simulink model "AnaModelFault000"  (R2018b)
settings: Solver=VariableStepAuto  StartTime=0.0  StopTime=2  MaxStep=1e-4  RelTol=1e-3
values from neighbouring files (symbols this model uses):
  J = 0.275e-3    (= 0.000275)    [StateSpace.m]    (also in init_AnaModel003.m)
  Ki = 1    [init_AnaModel003.m]
  Kp = 0.05    [init_AnaModel003.m]
  L0 = Ll + 1.5*Lms    (= 0.00130602)    [StateSpace.m]    (also in init_AnaModel003.m)
  L1 = Ll + 1.5*Lms    [AnaModel.m]    (also in StateSpace.m = (sqrt(3)* Llm + 1.5 *Lms); init_AnaModel003.m = (sqrt(3)* Llm + 1.5 *Lms))
  L2 = (sqrt(3)/2)*Lms + Llm    [AnaModel.m]    (also in StateSpace.m = 0.0010375; init_AnaModel003.m = 0.0010375)
  P = 6    [StateSpace.m]    (also in init_AnaModel003.m)
  Phi_f = 0.03    [StateSpace.m]    (also in init_AnaModel003.m)
  rs = 1.98    [StateSpace.m]    (also in init_AnaModel003.m)
  Tm = 1    [StateSpace.m]    (also in init_AnaModel003.m)
libraries: powerlib x46, powerlib_meascontrol x9, simulink x7
(part 1 of 2)
settings Model: Creator=admin  LastModifiedBy=aeish
settings SolverCC: ZeroCrossAlgorithm=Adaptive
settings DebuggingCC: MaxConsecutiveZCsMsg=none  LibraryContextMissingDiagnostic=none
settings SFSimCC: SimUseLocalCustomCode=off
settings RTWCC: RTWUseLocalCustomCode=off

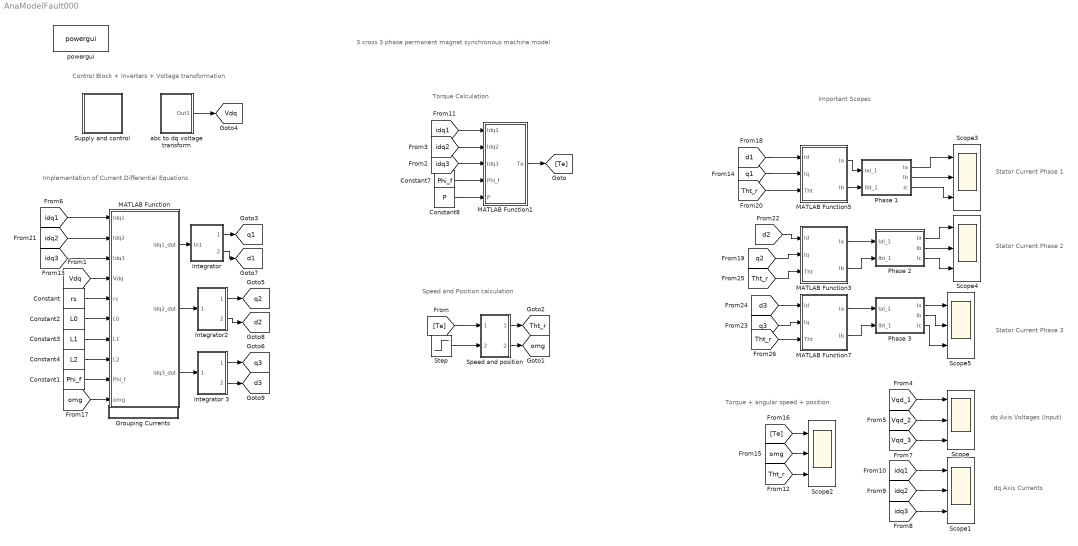
== system AnaModelFault000 ==
  note: 3 cross 3 phase permanent magnet synchronous machine model
  note: Torque + angular speed + position
  note: dq Axis Voltages (Input)
  note: Stator Current Phase 1
  note: Important Scopes
  note: Control Block + Inverters + Voltage transformation
  note: Speed and Position calculation
  note: Torque Calculation
  note: Implementation of Current Differential Equations
  note: Stator Current Phase 2
  note: Stator Current Phase 3
  note: dq Axis Currents
  Constant : Constant  Value=rs
  Constant1 : Constant  Value=Phi_f
  Constant2 : Constant  Value=L0
  Constant3 : Constant  Value=L1
  Constant4 : Constant  Value=L2
  Constant7 : Constant  Value=Phi_f
  Constant8 : Constant  Value=P
  Grouping Currents : Subsystem
  Integrator : Subsystem
  "Integrator 3 " : Subsystem
  "Integrator2 " : Subsystem
  MATLAB Function : MATLAB Function  TreatAsAtomicUnit=on
  MATLAB Function1 : MATLAB Function  TreatAsAtomicUnit=on
  MATLAB Function3 : MATLAB Function  TreatAsAtomicUnit=on
  MATLAB Function5 : MATLAB Function  TreatAsAtomicUnit=on
  MATLAB Function7 : MATLAB Function  TreatAsAtomicUnit=on
  Phase 1 : MATLAB Function  TreatAsAtomicUnit=on
  Phase 2 : MATLAB Function  TreatAsAtomicUnit=on
  Phase 3 : MATLAB Function  TreatAsAtomicUnit=on
  Scope{,1..5} (6 alike) : Scope  NumInputPorts=3
  Speed and position : Subsystem
  Step : Step  Time=0.05  After=Tm  SampleTime=0
  Supply and control : Subsystem
  abc to dq voltage transform : Subsystem
  powergui : powerlib/powergui  Priority=1  SimulationMode=Continuous  SampleTime=50e-6  frequency=60  Iterations=50  frequencyindice=0  Pbase=100e6  ErrMax=1e-4  UnitsV=kV  UnitsW=MW  buscounter=0  FunctionMessages=off  echomessages=off  EnableUseOfTLC=off  CurrentSourceSwitches=off  DisableSnubberDevices=off  DisableRonSwitches=off  DisableVfSwitches=off  DisplayEquations=off  SolverType=Tustin/Backward Euler (TBE)  Interpol=off  ExternalGateDelay=off  methode=off  Ts=100  x0status=blocks  SPID=on  SwTol=0  HookPort=off  RestoreLinks=warning  ResistiveCurrentMeasurement=off  Frange=[0:2:500]  Ylog=off  Xlog=on  ShowGrid=off  save=off  variable=ZData  structure=Vabc2  ZoomFFT=off  StartTime=0.2  cycles=1  DisplayStyle=1  fundamental=62  FreqAxis=on  MaxFrequency=1500  frequencyindicesteady=1  RmsSteady=1  display=off
      settings: SourceProductName=Simscape Electrical
  tag scope: Tht_r=global, Vdq=global, d1=global, d2=global, d3=global, omg=global, q1=global, q2=global, q3=global
  wires:
  Constant/1 -> MATLAB Function/5(rs)
  Constant3/1 -> MATLAB Function/7(L1)
  Constant2/1 -> MATLAB Function/6(L0)
  Constant4/1 -> MATLAB Function/8(L2)
  Constant1/1 -> MATLAB Function/9(Phi_f)
  [idq2] -> MATLAB Function/2(Idq2)
  [idq1] -> MATLAB Function/1(Idq1)
  [Vdq] -> MATLAB Function/4(Vdq)
  [omg] -> MATLAB Function/10(omg)
  [Vqd_1] -> Scope/1
  [Vqd_2] -> Scope/2
  [Vqd_3] -> Scope/3
  [idq1] -> Scope1/1
  [idq2] -> Scope1/2
  [idq3] -> Scope1/3
  abc to dq voltage transform/1(Out1) -> [Vdq]
  MATLAB Function/1(idq1_dot) -> Integrator/1(In1)
  Integrator/1(Out1) -> [q1]
  Integrator/2(Out2) -> [d1]
  MATLAB Function/2(idq2_dot) -> "Integrator2 "/1(In1)
  "Integrator2 "/1(Out1) -> [q2]
  "Integrator2 "/2(Out2) -> [d2]
  MATLAB Function/3(idq3_dot) -> "Integrator 3 "/1(In1)
  "Integrator 3 "/1(Out1) -> [q3]
  "Integrator 3 "/2(Out2) -> [d3]
  [idq1] -> MATLAB Function1/1(Idq1)
  [idq2] -> MATLAB Function1/2(Idq2)
  [idq3] -> MATLAB Function1/3(Idq3)
  Constant7/1 -> MATLAB Function1/4(Phi_f)
  Constant8/1 -> MATLAB Function1/5(P)
  MATLAB Function1/1(Te) -> [Te]
  [Tht_r] -> Scope2/3
  [omg] -> Scope2/2
  [Te] -> Scope2/1
  [Te] -> Speed and position/1(In1)
  Step/1 -> Speed and position/2(In2)
  Speed and position/1(Out1) -> [Tht_r]
  Speed and position/2(Out2) -> [omg]
  MATLAB Function5/1(Ia) -> Phase 1/1(Ial_1)
  Phase 1/1(Ia) -> Scope3/1
  Phase 1/2(Ib) -> Scope3/2
  Phase 1/3(Ic) -> Scope3/3
  [Tht_r] -> MATLAB Function5/3(Tht)
  MATLAB Function5/2(Ib) -> Phase 1/2(Ibt_1)
  [idq3] -> MATLAB Function/3(Idq3)
  [q1] -> MATLAB Function5/2(Iq)
  [d1] -> MATLAB Function5/1(Id)
  MATLAB Function7/1(Ia) -> Phase 3/1(Ial_1)
  MATLAB Function7/2(Ib) -> Phase 3/2(Ibt_1)
  Phase 2/1(Ia) -> Scope4/1
  Phase 2/2(Ib) -> Scope4/2
  Phase 2/3(Ic) -> Scope4/3
  Phase 3/1(Ia) -> Scope5/1
  Phase 3/2(Ib) -> Scope5/2
  Phase 3/3(Ic) -> Scope5/3
  MATLAB Function3/1(Ia) -> Phase 2/1(Ial_1)
  MATLAB Function3/2(Ib) -> Phase 2/2(Ibt_1)
  [q2] -> MATLAB Function3/2(Iq)
  [d2] -> MATLAB Function3/1(Id)
  [q3] -> MATLAB Function7/2(Iq)
  [d3] -> MATLAB Function7/1(Id)
  [Tht_r] -> MATLAB Function3/3(Tht)
  [Tht_r] -> MATLAB Function7/3(Tht)

== system AnaModelFault000/Grouping Currents ==
  Mux3 : Mux  Inputs=2
  Mux4 : Mux  Inputs=2
  Mux5 : Mux  Inputs=2
  tag scope: idq1=global, idq2=global, idq3=global
  wires:
  Mux5/1 -> [idq3]
  Mux3/1 -> [idq1]
  [d1] -> Mux3/2
  [q1] -> Mux3/1
  [d3] -> Mux5/2
  [q3] -> Mux5/1
  Mux4/1 -> [idq2]
  [q2] -> Mux4/1
  [d2] -> Mux4/2

== system AnaModelFault000/Integrator ==
  In1 : Inport
  Demux : Demux  Outputs=2
  Integrator : Integrator
  Integrator1 : Integrator
  Out1 : Outport
  Out2 : Outport  Port=2
  wires:
  Demux/2 -> Integrator1/1
  Integrator/1 -> Out1/1
  Integrator1/1 -> Out2/1
  In1/1 -> Demux/1
  Demux/1 -> Integrator/1

== system AnaModelFault000/Integrator 3  ==
  In1 : Inport
  Demux2 : Demux  Outputs=2
  Integrator4 : Integrator
  Integrator5 : Integrator
  Out1 : Outport
  Out2 : Outport  Port=2
  wires:
  Demux2/1 -> Integrator4/1
  Integrator5/1 -> Out2/1
  Demux2/2 -> Integrator5/1
  In1/1 -> Demux2/1
  Integrator4/1 -> Out1/1

== system AnaModelFault000/Integrator2  ==
  In1 : Inport
  Demux1 : Demux  Outputs=2
  Integrator2 : Integrator
  Integrator3 : Integrator
  Out1 : Outport
  Out2 : Outport  Port=2
  wires:
  Demux1/2 -> Integrator3/1
  Integrator3/1 -> Out2/1
  Integrator2/1 -> Out1/1
  In1/1 -> Demux1/1
  Demux1/1 -> Integrator2/1

== system AnaModelFault000/Speed and position ==
  In1 : Inport
  In2 : Inport  Port=2
  Constant9 : Constant  Value=-1/J
  Integrator1 : Integrator
  Integrator2 : Integrator  WrapState=on
  Product1 : Product
  Sum : Sum  Inputs=+-
  Out1 : Outport
  Out2 : Outport  Port=2
  wires:
  Integrator2/1 -> Out1/1
  In2/1 -> Sum/2
  Product1/1 -> Integrator1/1
  Constant9/1 -> Product1/2
  In1/1 -> Sum/1
  Sum/1 -> Product1/1
  Integrator1/1 -> Out2/1, Integrator2/1

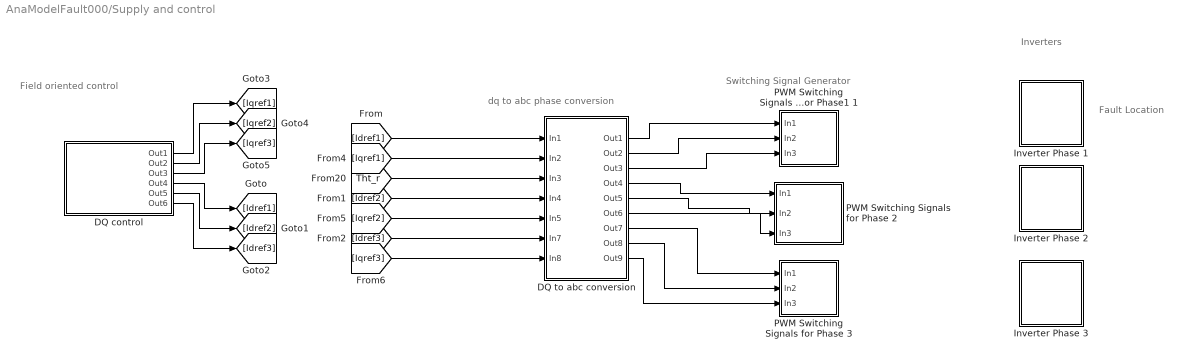
== system AnaModelFault000/Supply and control ==
  note: Fault Location
  note: Inverters
  note: Field oriented control
  note: dq to abc phase conversion
  note: Switching Signal Generator
  DQ control : Subsystem
  "DQ to abc conversion " : Subsystem
  "Inverter Phase 1 " : Subsystem
  Inverter Phase 2 : Subsystem
  Inverter Phase 3 : Subsystem
  PWM Switching Signals for Phase 2 : Subsystem
  "PWM Switching Signals for Phase 3 " : Subsystem
  PWM Switching Signals for Phase1 1 : Subsystem
  wires:
  DQ control/1(Out1) -> [Iqref1]
  DQ control/2(Out2) -> [Iqref2]
  DQ control/3(Out3) -> [Iqref3]
  DQ control/4(Out4) -> [Idref1]
  DQ control/5(Out5) -> [Idref2]
  DQ control/6(Out6) -> [Idref3]
  [Idref1] -> "DQ to abc conversion "/1(In1)
  [Iqref1] -> "DQ to abc conversion "/2(In2)
  [Tht_r] -> "DQ to abc conversion "/3(In3)
  [Idref2] -> "DQ to abc conversion "/4(In4)
  [Iqref2] -> "DQ to abc conversion "/5(In5)
  [Idref3] -> "DQ to abc conversion "/6(In7)
  [Iqref3] -> "DQ to abc conversion "/7(In8)
  "DQ to abc conversion "/1(Out1) -> PWM Switching Signals for Phase1 1/1(In1)
  "DQ to abc conversion "/2(Out2) -> PWM Switching Signals for Phase1 1/2(In2)
  "DQ to abc conversion "/3(Out3) -> PWM Switching Signals for Phase1 1/3(In3)
  "DQ to abc conversion "/4(Out4) -> PWM Switching Signals for Phase 2/1(In1)
  "DQ to abc conversion "/5(Out5) -> PWM Switching Signals for Phase 2/2(In2)
  "DQ to abc conversion "/6(Out6) -> PWM Switching Signals for Phase 2/3(In3)
  "DQ to abc conversion "/7(Out7) -> "PWM Switching Signals for Phase 3 "/1(In1)
  "DQ to abc conversion "/8(Out8) -> "PWM Switching Signals for Phase 3 "/2(In2)
  "DQ to abc conversion "/9(Out9) -> "PWM Switching Signals for Phase 3 "/3(In3)

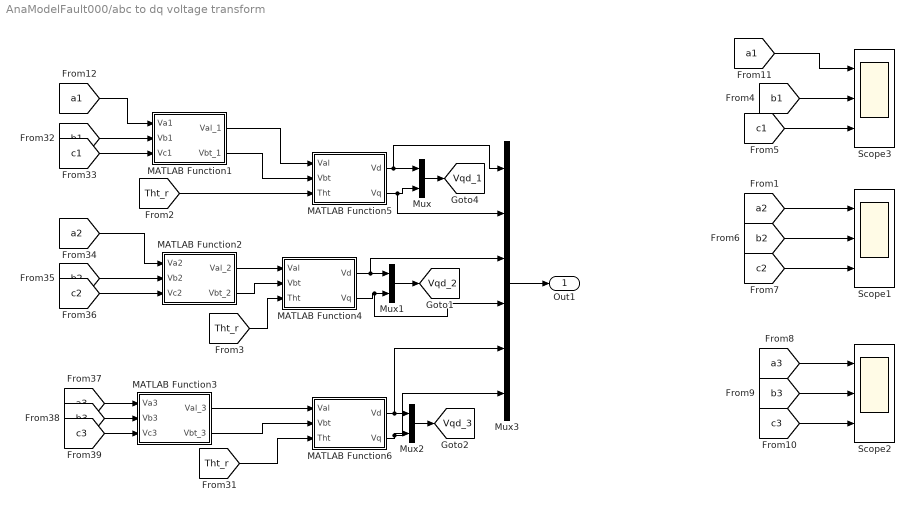
== system AnaModelFault000/abc to dq voltage transform ==
  MATLAB Function1 : MATLAB Function  TreatAsAtomicUnit=on
  MATLAB Function2 : MATLAB Function  TreatAsAtomicUnit=on
  MATLAB Function3 : MATLAB Function  TreatAsAtomicUnit=on
  MATLAB Function4 : MATLAB Function  TreatAsAtomicUnit=on
  MATLAB Function5 : MATLAB Function  TreatAsAtomicUnit=on
  MATLAB Function6 : MATLAB Function  TreatAsAtomicUnit=on
  Mux : Mux  Inputs=2
  Mux1 : Mux  Inputs=2
  Mux2 : Mux  Inputs=2
  Mux3 : Mux  Inputs=6
  Scope1 : Scope  NumInputPorts=3
  Scope2 : Scope  NumInputPorts=3
  Scope3 : Scope  NumInputPorts=3
  Out1 : Outport
  tag scope: Vqd_1=global, Vqd_2=global, Vqd_3=global
  wires:
  MATLAB Function6/1(Vd) -> Mux3/5, Mux2/1
  MATLAB Function1/2(Vbt_1) -> MATLAB Function5/2(Vbt)
  MATLAB Function4/1(Vd) -> Mux3/3, Mux1/1
  [Tht_r] -> MATLAB Function6/3(Tht)
  MATLAB Function4/2(Vq) -> Mux3/4, Mux1/2
  Mux1/1 -> [Vqd_2]
  Mux/1 -> [Vqd_1]
  MATLAB Function6/2(Vq) -> Mux3/6, Mux2/2
  MATLAB Function2/1(Val_2) -> MATLAB Function4/1(Val)
  [a3] -> MATLAB Function3/1(Va3)
  [Tht_r] -> MATLAB Function5/3(Tht)
  MATLAB Function2/2(Vbt_2) -> MATLAB Function4/2(Vbt)
  [b1] -> MATLAB Function1/2(Vb1)
  MATLAB Function5/1(Vd) -> Mux3/1, Mux/1
  [Tht_r] -> MATLAB Function4/3(Tht)
  Mux2/1 -> [Vqd_3]
  MATLAB Function3/2(Vbt_3) -> MATLAB Function6/2(Vbt)
  [b3] -> MATLAB Function3/2(Vb3)
  MATLAB Function5/2(Vq) -> Mux3/2, Mux/2
  MATLAB Function3/1(Val_3) -> MATLAB Function6/1(Val)
  [c2] -> MATLAB Function2/3(Vc2)
  [b2] -> MATLAB Function2/2(Vb2)
  Mux3/1 -> Out1/1
  [a2] -> MATLAB Function2/1(Va2)
  [c1] -> MATLAB Function1/3(Vc1)
  [c3] -> MATLAB Function3/3(Vc3)
  MATLAB Function1/1(Val_1) -> MATLAB Function5/1(Val)
  [c1] -> Scope3/3
  [b1] -> Scope3/2
  [a1] -> Scope3/1
  [a2] -> Scope1/1
  [b2] -> Scope1/2
  [c2] -> Scope1/3
  [a3] -> Scope2/1
  [c3] -> Scope2/3
  [b3] -> Scope2/2
  [a1] -> MATLAB Function1/1(Va1)

== system AnaModelFault000/Supply and control/DQ control ==
  Direct Axis Control : Subsystem
  "Q axis Control " : Subsystem
  Out1 : Outport
  Out2 : Outport  Port=2
  Out3 : Outport  Port=3
  Out4 : Outport  Port=4
  Out5 : Outport  Port=5
  Out6 : Outport  Port=6
  wires:
  Direct Axis Control/3(Out3) -> Out6/1
  Direct Axis Control/2(Out2) -> Out5/1
  "Q axis Control "/1(Out1) -> Out1/1
  "Q axis Control "/2(Out2) -> Out2/1
  Direct Axis Control/1(Out1) -> Out4/1
  "Q axis Control "/3(Out3) -> Out3/1

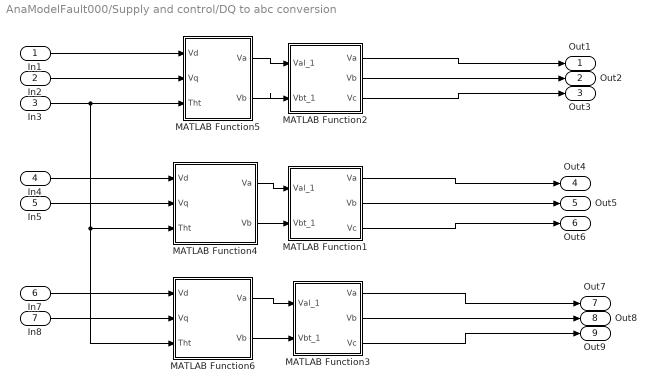
== system AnaModelFault000/Supply and control/DQ to abc conversion  ==
  In1 : Inport
  In2 : Inport  Port=2
  In3 : Inport  Port=3
  In4 : Inport  Port=4
  In5 : Inport  Port=5
  In7 : Inport  Port=6
  In8 : Inport  Port=7
  MATLAB Function1 : MATLAB Function  TreatAsAtomicUnit=on
  MATLAB Function2 : MATLAB Function  TreatAsAtomicUnit=on
  MATLAB Function3 : MATLAB Function  TreatAsAtomicUnit=on
  MATLAB Function4 : MATLAB Function  TreatAsAtomicUnit=on
  MATLAB Function5 : MATLAB Function  TreatAsAtomicUnit=on
  MATLAB Function6 : MATLAB Function  TreatAsAtomicUnit=on
  Out1 : Outport
  Out2 : Outport  Port=2
  Out3 : Outport  Port=3
  Out4 : Outport  Port=4
  Out5 : Outport  Port=5
  Out6 : Outport  Port=6
  Out7 : Outport  Port=7
  Out8 : Outport  Port=8
  Out9 : Outport  Port=9
  wires:
  MATLAB Function6/1(Va) -> MATLAB Function3/1(Val_1)
  MATLAB Function5/1(Va) -> MATLAB Function2/1(Val_1)
  MATLAB Function6/2(Vb) -> MATLAB Function3/2(Vbt_1)
  MATLAB Function5/2(Vb) -> MATLAB Function2/2(Vbt_1)
  MATLAB Function1/2(Vb) -> Out5/1
  MATLAB Function2/1(Va) -> Out1/1
  MATLAB Function4/2(Vb) -> MATLAB Function1/2(Vbt_1)
  MATLAB Function4/1(Va) -> MATLAB Function1/1(Val_1)
  In1/1 -> MATLAB Function5/1(Vd)
  MATLAB Function2/2(Vb) -> Out2/1
  MATLAB Function2/3(Vc) -> Out3/1
  In4/1 -> MATLAB Function4/1(Vd)
  In7/1 -> MATLAB Function6/1(Vd)
  In3/1 -> MATLAB Function6/3(Tht), MATLAB Function4/3(Tht), MATLAB Function5/3(Tht)
  MATLAB Function3/1(Va) -> Out7/1
  MATLAB Function3/3(Vc) -> Out9/1
  In8/1 -> MATLAB Function6/2(Vq)
  MATLAB Function3/2(Vb) -> Out8/1
  MATLAB Function1/1(Va) -> Out4/1
  MATLAB Function1/3(Vc) -> Out6/1
  In2/1 -> MATLAB Function5/2(Vq)
  In5/1 -> MATLAB Function4/2(Vq)

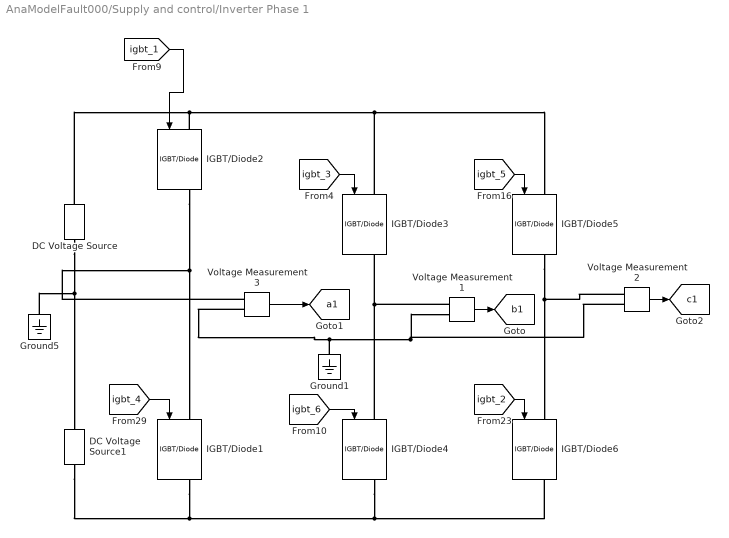
== system AnaModelFault000/Supply and control/Inverter Phase 1  ==
  DC Voltage Source : powerlib/Electrical Sources/DC Voltage Source  Amplitude=230*sqrt(2)  Measurements=None
      settings: SourceProductName=Simscape Electrical
  DC Voltage Source1 : powerlib/Electrical Sources/DC Voltage Source  Amplitude=230*sqrt(2)  Measurements=None
      settings: SourceProductName=Simscape Electrical
  Ground1 : powerlib/Elements/Ground  LConnTagsString=a
      settings: SourceProductName=Simscape Electrical
  Ground5 : powerlib/Elements/Ground  LConnTagsString=a
      settings: SourceProductName=Simscape Electrical
  IGBT/Diode{1..6} (6 alike) : powerlib/Power Electronics/IGBT//Diode  Ron=1e-3  Rs=1e5  Cs=inf  Measurements=on
      settings: SourceProductName=Simscape Electrical
  Voltage Measurement1 : powerlib/Measurements/Voltage Measurement  PhasorSimulation=off  OutputType=Complex  PSBequivalent=0
      settings: SourceProductName=Simscape Electrical
  Voltage Measurement2 : powerlib/Measurements/Voltage Measurement  PhasorSimulation=off  OutputType=Complex  PSBequivalent=0
      settings: SourceProductName=Simscape Electrical
  Voltage Measurement3 : powerlib/Measurements/Voltage Measurement  PhasorSimulation=off  OutputType=Complex  PSBequivalent=0
      settings: SourceProductName=Simscape Electrical
  tag scope: a1=global, b1=global, c1=global
  wires:
  Voltage Measurement2/1 -> [c1]
  [igbt_3] -> IGBT/Diode3/1
  [igbt_6] -> IGBT/Diode4/1
  Voltage Measurement3/1 -> [a1]
  [igbt_4] -> IGBT/Diode1/1
  [igbt_5] -> IGBT/Diode5/1
  [igbt_2] -> IGBT/Diode6/1
  Voltage Measurement1/1 -> [b1]
  [igbt_1] -> IGBT/Diode2/1
  connections:
  IGBT/Diode4/LConn1 -- Voltage Measurement1/LConn1 -- IGBT/Diode3/RConn1
  IGBT/Diode1/RConn1 -- DC Voltage Source1/LConn1 -- IGBT/Diode4/RConn1 -- IGBT/Diode6/RConn1
  IGBT/Diode5/RConn1 -- Voltage Measurement2/LConn1 -- IGBT/Diode6/LConn1
  IGBT/Diode2/LConn1 -- DC Voltage Source/RConn1 -- IGBT/Diode3/LConn1 -- IGBT/Diode5/LConn1
  DC Voltage Source/LConn1 -- Ground5/LConn1 -- DC Voltage Source1/RConn1
  IGBT/Diode2/RConn1 -- Voltage Measurement3/LConn1 -- IGBT/Diode1/LConn1
  Ground1/LConn1 -- Voltage Measurement3/LConn2 -- Voltage Measurement2/LConn2 -- Voltage Measurement1/LConn2

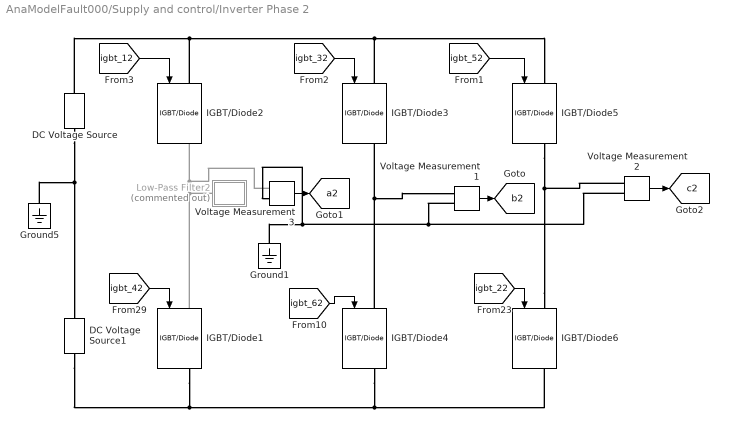
== system AnaModelFault000/Supply and control/Inverter Phase 2 ==
  DC Voltage Source : powerlib/Electrical Sources/DC Voltage Source  Amplitude=230*sqrt(2)  Measurements=None
      settings: SourceProductName=Simscape Electrical
  DC Voltage Source1 : powerlib/Electrical Sources/DC Voltage Source  Amplitude=230*sqrt(2)  Measurements=None
      settings: SourceProductName=Simscape Electrical
  Ground1 : powerlib/Elements/Ground  LConnTagsString=a
      settings: SourceProductName=Simscape Electrical
  Ground5 : powerlib/Elements/Ground  LConnTagsString=a
      settings: SourceProductName=Simscape Electrical
  IGBT/Diode{1..6} (6 alike) : powerlib/Power Electronics/IGBT//Diode  Ron=1e-3  Rs=1e5  Cs=inf  Measurements=on
      settings: SourceProductName=Simscape Electrical
  Low-Pass Filter2 : Subsystem  Commented=on
  Voltage Measurement1 : powerlib/Measurements/Voltage Measurement  PhasorSimulation=off  OutputType=Complex  PSBequivalent=0
      settings: SourceProductName=Simscape Electrical
  Voltage Measurement2 : powerlib/Measurements/Voltage Measurement  PhasorSimulation=off  OutputType=Complex  PSBequivalent=0
      settings: SourceProductName=Simscape Electrical
  Voltage Measurement3 : powerlib/Measurements/Voltage Measurement  PhasorSimulation=off  OutputType=Complex  PSBequivalent=0
      settings: SourceProductName=Simscape Electrical
  tag scope: a2=global, b2=global, c2=global
  wires:
  Voltage Measurement1/1 -> [b2]
  [igbt_22] -> IGBT/Diode6/1
  [igbt_42] -> IGBT/Diode1/1
  Voltage Measurement3/1 -> [a2]
  [igbt_62] -> IGBT/Diode4/1
  Voltage Measurement2/1 -> [c2]
  [igbt_12] -> IGBT/Diode2/1
  [igbt_32] -> IGBT/Diode3/1
  [igbt_52] -> IGBT/Diode5/1
  connections:
  IGBT/Diode3/RConn1 -- Voltage Measurement1/LConn1 -- IGBT/Diode4/LConn1
  Low-Pass Filter2/LConn1 -- Voltage Measurement3/LConn1 -- IGBT/Diode2/RConn1 -- IGBT/Diode1/LConn1
  Ground5/LConn1 -- DC Voltage Source/LConn1 -- DC Voltage Source1/RConn1
  IGBT/Diode3/LConn1 -- IGBT/Diode2/LConn1 -- DC Voltage Source/RConn1 -- IGBT/Diode5/LConn1
  IGBT/Diode6/LConn1 -- Voltage Measurement2/LConn1 -- IGBT/Diode5/RConn1
  DC Voltage Source1/LConn1 -- IGBT/Diode1/RConn1 -- IGBT/Diode6/RConn1 -- IGBT/Diode4/RConn1
  Ground1/LConn1 -- Voltage Measurement1/LConn2 -- Voltage Measurement2/LConn2 -- Voltage Measurement3/LConn2

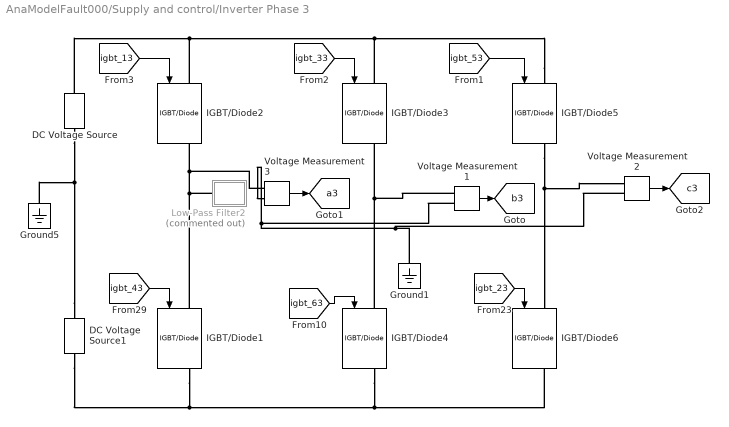
== system AnaModelFault000/Supply and control/Inverter Phase 3 ==
  DC Voltage Source : powerlib/Electrical Sources/DC Voltage Source  Amplitude=230*sqrt(2)  Measurements=None
      settings: SourceProductName=Simscape Electrical
  DC Voltage Source1 : powerlib/Electrical Sources/DC Voltage Source  Amplitude=230*sqrt(2)  Measurements=None
      settings: SourceProductName=Simscape Electrical
  Ground1 : powerlib/Elements/Ground  LConnTagsString=a
      settings: SourceProductName=Simscape Electrical
  Ground5 : powerlib/Elements/Ground  LConnTagsString=a
      settings: SourceProductName=Simscape Electrical
  IGBT/Diode{1..6} (6 alike) : powerlib/Power Electronics/IGBT//Diode  Ron=1e-3  Rs=1e5  Cs=inf  Measurements=on
      settings: SourceProductName=Simscape Electrical
  Low-Pass Filter2 : Subsystem  Commented=on
  Voltage Measurement1 : powerlib/Measurements/Voltage Measurement  PhasorSimulation=off  OutputType=Complex  PSBequivalent=0
      settings: SourceProductName=Simscape Electrical
  Voltage Measurement2 : powerlib/Measurements/Voltage Measurement  PhasorSimulation=off  OutputType=Complex  PSBequivalent=0
      settings: SourceProductName=Simscape Electrical
  Voltage Measurement3 : powerlib/Measurements/Voltage Measurement  PhasorSimulation=off  OutputType=Complex  PSBequivalent=0
      settings: SourceProductName=Simscape Electrical
  tag scope: a3=global, b3=global, c3=global
  wires:
  [igbt_53] -> IGBT/Diode5/1
  [igbt_33] -> IGBT/Diode3/1
  [igbt_13] -> IGBT/Diode2/1
  Voltage Measurement2/1 -> [c3]
  [igbt_63] -> IGBT/Diode4/1
  Voltage Measurement3/1 -> [a3]
  [igbt_43] -> IGBT/Diode1/1
  [igbt_23] -> IGBT/Diode6/1
  Voltage Measurement1/1 -> [b3]
  connections:
  IGBT/Diode4/LConn1 -- Voltage Measurement1/LConn1 -- IGBT/Diode3/RConn1
  IGBT/Diode4/RConn1 -- IGBT/Diode6/RConn1 -- IGBT/Diode1/RConn1 -- DC Voltage Source1/LConn1
  IGBT/Diode5/LConn1 -- DC Voltage Source/RConn1 -- IGBT/Diode2/LConn1 -- IGBT/Diode3/LConn1
  DC Voltage Source1/RConn1 -- DC Voltage Source/LConn1 -- Ground5/LConn1
  IGBT/Diode1/LConn1 -- Voltage Measurement3/LConn1 -- IGBT/Diode2/RConn1 -- Low-Pass Filter2/LConn1
  IGBT/Diode5/RConn1 -- Voltage Measurement2/LConn1 -- IGBT/Diode6/LConn1
  Ground1/LConn1 -- Voltage Measurement2/LConn2 -- Voltage Measurement1/LConn2 -- Voltage Measurement3/LConn2

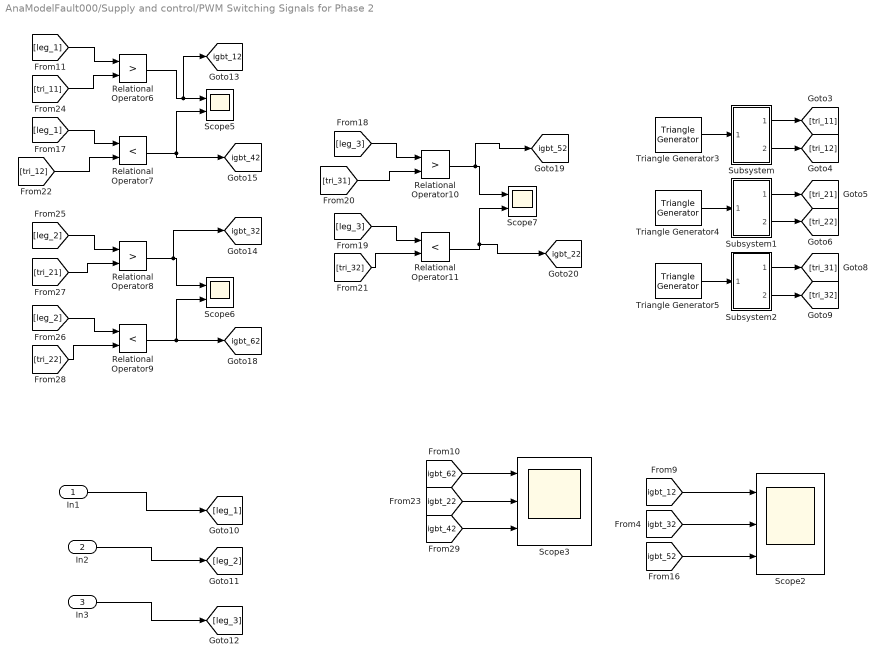
== system AnaModelFault000/Supply and control/PWM Switching Signals for Phase 2 ==
  In1 : Inport
  In2 : Inport  Port=2
  In3 : Inport  Port=3
  Relational Operator10 : RelationalOperator  Operator=>  OutDataTypeStr=boolean  RndMeth=Simplest
  Relational Operator11 : RelationalOperator  Operator=<  OutDataTypeStr=boolean  RndMeth=Simplest
  Relational Operator6 : RelationalOperator  Operator=>  OutDataTypeStr=boolean  RndMeth=Simplest
  Relational Operator7 : RelationalOperator  Operator=<  OutDataTypeStr=boolean  RndMeth=Simplest
  Relational Operator8 : RelationalOperator  Operator=>  OutDataTypeStr=boolean  RndMeth=Simplest
  Relational Operator9 : RelationalOperator  Operator=<  OutDataTypeStr=boolean  RndMeth=Simplest
  Scope2 : Scope  NumInputPorts=3
  Scope3 : Scope  NumInputPorts=3
  Scope5 : Scope  NumInputPorts=2
  Scope6 : Scope  NumInputPorts=2
  Scope7 : Scope  NumInputPorts=2
  Subsystem : Subsystem
  Subsystem1 : Subsystem
  Subsystem2 : Subsystem
  Triangle Generator3 : powerlib_meascontrol/Pulse & Signal Generators/Triangle Generator  Freq=10e3  Phase=-30  Ts=0
      settings: SourceProductName=Simscape Electrical
  Triangle Generator4 : powerlib_meascontrol/Pulse & Signal Generators/Triangle Generator  Freq=10e3  Phase=-30-120  Ts=0
      settings: SourceProductName=Simscape Electrical
  Triangle Generator5 : powerlib_meascontrol/Pulse & Signal Generators/Triangle Generator  Freq=10e3  Phase=+30+120  Ts=0
      settings: SourceProductName=Simscape Electrical
  tag scope: igbt_12=global, igbt_22=global, igbt_32=global, igbt_42=global, igbt_52=global, igbt_62=global
  wires:
  [igbt_42] -> Scope3/3
  [igbt_12] -> Scope2/1
  [igbt_62] -> Scope3/1
  [igbt_32] -> Scope2/2
  [igbt_52] -> Scope2/3
  [igbt_22] -> Scope3/2
  In3/1 -> [leg_3]
  In2/1 -> [leg_2]
  In1/1 -> [leg_1]
  Relational Operator8/1 -> [igbt_32], Scope6/1
  Relational Operator9/1 -> [igbt_62], Scope6/2
  Relational Operator11/1 -> [igbt_22], Scope7/2
  Relational Operator6/1 -> [igbt_12], Scope5/1
  [tri_12] -> Relational Operator7/2
  [leg_3] -> Relational Operator10/1
  [tri_32] -> Relational Operator11/2
  [leg_1] -> Relational Operator7/1
  [tri_22] -> Relational Operator9/2
  Relational Operator7/1 -> [igbt_42], Scope5/2
  [tri_21] -> Relational Operator8/2
  [tri_11] -> Relational Operator6/2
  Relational Operator10/1 -> [igbt_52], Scope7/1
  [leg_2] -> Relational Operator9/1
  [tri_31] -> Relational Operator10/2
  [leg_1] -> Relational Operator6/1
  [leg_3] -> Relational Operator11/1
  [leg_2] -> Relational Operator8/1
  Triangle Generator4/1 -> Subsystem1/1(In1)
  Triangle Generator3/1 -> Subsystem/1(In1)
  Subsystem1/1(Out1) -> [tri_21]
  Subsystem/2(Out2) -> [tri_12]
  Subsystem2/1(Out1) -> [tri_31]
  Subsystem/1(Out1) -> [tri_11]
  Subsystem2/2(Out2) -> [tri_32]
  Triangle Generator5/1 -> Subsystem2/1(In1)
  Subsystem1/2(Out2) -> [tri_22]

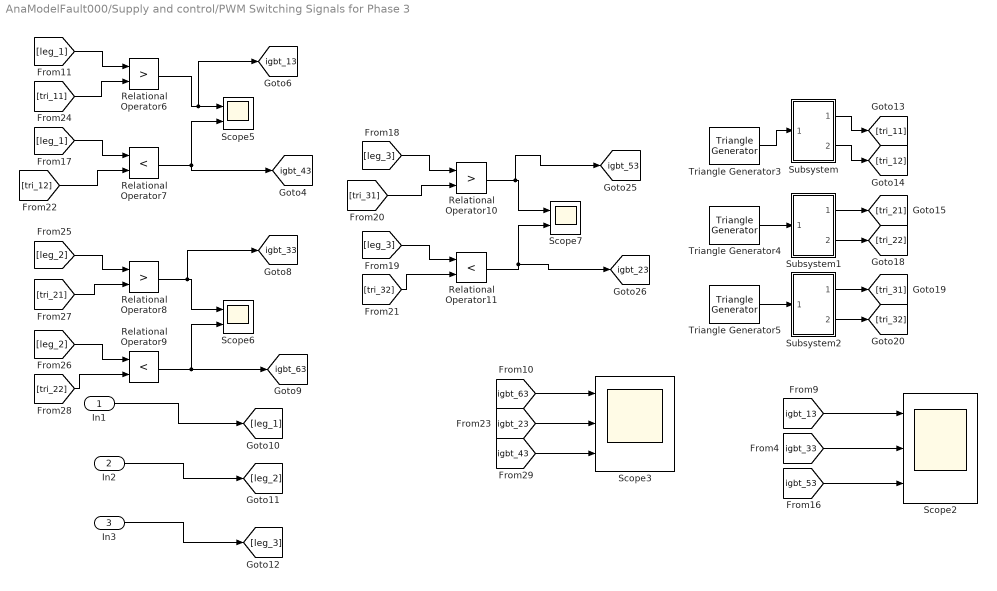
== system AnaModelFault000/Supply and control/PWM Switching Signals for Phase 3  ==
  In1 : Inport
  In2 : Inport  Port=2
  In3 : Inport  Port=3
  Relational Operator10 : RelationalOperator  Operator=>  OutDataTypeStr=boolean  RndMeth=Simplest
  Relational Operator11 : RelationalOperator  Operator=<  OutDataTypeStr=boolean  RndMeth=Simplest
  Relational Operator6 : RelationalOperator  Operator=>  OutDataTypeStr=boolean  RndMeth=Simplest
  Relational Operator7 : RelationalOperator  Operator=<  OutDataTypeStr=boolean  RndMeth=Simplest
  Relational Operator8 : RelationalOperator  Operator=>  OutDataTypeStr=boolean  RndMeth=Simplest
  Relational Operator9 : RelationalOperator  Operator=<  OutDataTypeStr=boolean  RndMeth=Simplest
  Scope2 : Scope  NumInputPorts=3
  Scope3 : Scope  NumInputPorts=3
  Scope5 : Scope  NumInputPorts=2
  Scope6 : Scope  NumInputPorts=2
  Scope7 : Scope  NumInputPorts=2
  Subsystem : Subsystem
  Subsystem1 : Subsystem
  Subsystem2 : Subsystem
  Triangle Generator3 : powerlib_meascontrol/Pulse & Signal Generators/Triangle Generator  Freq=10e3  Phase=-60  Ts=0
      settings: SourceProductName=Simscape Electrical
  Triangle Generator4 : powerlib_meascontrol/Pulse & Signal Generators/Triangle Generator  Freq=10e3  Phase=-120-60  Ts=0
      settings: SourceProductName=Simscape Electrical
  Triangle Generator5 : powerlib_meascontrol/Pulse & Signal Generators/Triangle Generator  Freq=10e3  Phase=120+60  Ts=0
      settings: SourceProductName=Simscape Electrical
  tag scope: igbt_13=global, igbt_23=global, igbt_33=global, igbt_43=global, igbt_53=global, igbt_63=global
  wires:
  [igbt_23] -> Scope3/2
  [igbt_53] -> Scope2/3
  [igbt_33] -> Scope2/2
  [igbt_63] -> Scope3/1
  [igbt_13] -> Scope2/1
  [igbt_43] -> Scope3/3
  In3/1 -> [leg_3]
  In2/1 -> [leg_2]
  In1/1 -> [leg_1]
  Triangle Generator4/1 -> Subsystem1/1(In1)
  Triangle Generator3/1 -> Subsystem/1(In1)
  Subsystem1/1(Out1) -> [tri_21]
  Subsystem/2(Out2) -> [tri_12]
  Subsystem2/1(Out1) -> [tri_31]
  Subsystem/1(Out1) -> [tri_11]
  Subsystem2/2(Out2) -> [tri_32]
  Triangle Generator5/1 -> Subsystem2/1(In1)
  Subsystem1/2(Out2) -> [tri_22]
  [leg_1] -> Relational Operator6/1
  [leg_3] -> Relational Operator11/1
  [leg_2] -> Relational Operator8/1
  [leg_2] -> Relational Operator9/1
  [tri_11] -> Relational Operator6/2
  Relational Operator10/1 -> [igbt_53], Scope7/1
  Relational Operator7/1 -> [igbt_43], Scope5/2
  [leg_1] -> Relational Operator7/1
  [tri_31] -> Relational Operator10/2
  [tri_32] -> Relational Operator11/2
  [tri_12] -> Relational Operator7/2
  Relational Operator6/1 -> [igbt_13], Scope5/1
  [tri_22] -> Relational Operator9/2
  Relational Operator8/1 -> [igbt_33], Scope6/1
  Relational Operator9/1 -> [igbt_63], Scope6/2
  [tri_21] -> Relational Operator8/2
  Relational Operator11/1 -> [igbt_23], Scope7/2
  [leg_3] -> Relational Operator10/1

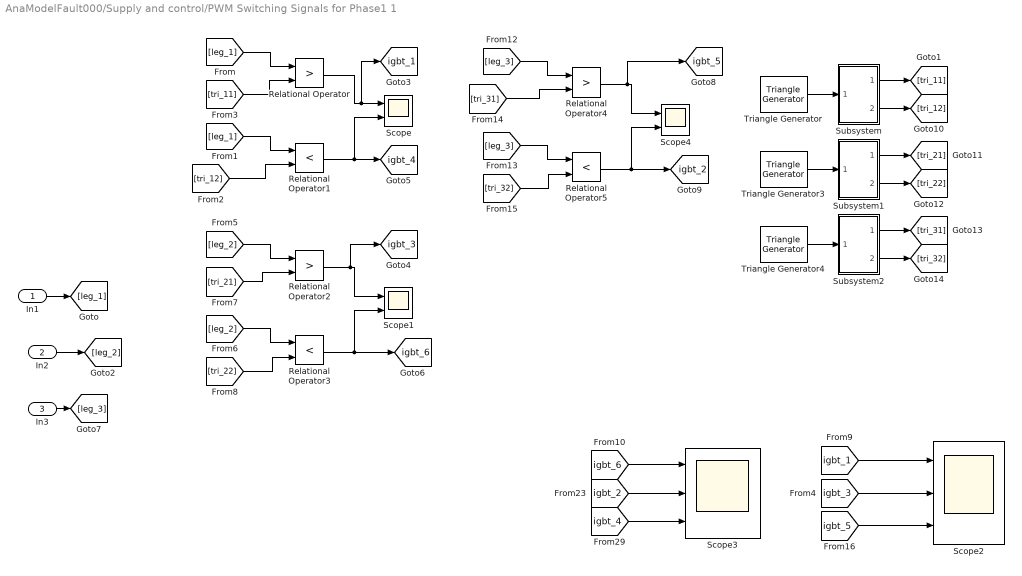
== system AnaModelFault000/Supply and control/PWM Switching Signals for Phase1 1 ==
  In1 : Inport
  In2 : Inport  Port=2
  In3 : Inport  Port=3
  Relational Operator : RelationalOperator  Operator=>  OutDataTypeStr=boolean  RndMeth=Simplest
  Relational Operator1 : RelationalOperator  Operator=<  OutDataTypeStr=boolean  RndMeth=Simplest
  Relational Operator2 : RelationalOperator  Operator=>  OutDataTypeStr=boolean  RndMeth=Simplest
  Relational Operator3 : RelationalOperator  Operator=<  OutDataTypeStr=boolean  RndMeth=Simplest
  Relational Operator4 : RelationalOperator  Operator=>  OutDataTypeStr=boolean  RndMeth=Simplest
  Relational Operator5 : RelationalOperator  Operator=<  OutDataTypeStr=boolean  RndMeth=Simplest
  Scope : Scope  NumInputPorts=2
  Scope1 : Scope  NumInputPorts=2
  Scope2 : Scope  NumInputPorts=3
  Scope3 : Scope  NumInputPorts=3
  Scope4 : Scope  NumInputPorts=2
  Subsystem : Subsystem
  Subsystem1 : Subsystem
  Subsystem2 : Subsystem
  Triangle Generator : powerlib_meascontrol/Pulse & Signal Generators/Triangle Generator  Freq=10e3  Phase=0  Ts=0
      settings: SourceProductName=Simscape Electrical
  Triangle Generator3 : powerlib_meascontrol/Pulse & Signal Generators/Triangle Generator  Freq=10e3  Phase=-120  Ts=0
      settings: SourceProductName=Simscape Electrical
  Triangle Generator4 : powerlib_meascontrol/Pulse & Signal Generators/Triangle Generator  Freq=10e3  Phase=120  Ts=0
      settings: SourceProductName=Simscape Electrical
  tag scope: igbt_1=global, igbt_2=global, igbt_3=global, igbt_4=global, igbt_5=global, igbt_6=global
  wires:
  [tri_31] -> Relational Operator4/2
  [tri_21] -> Relational Operator2/2
  [igbt_2] -> Scope3/2
  Relational Operator4/1 -> [igbt_5], Scope4/1
  [leg_3] -> Relational Operator4/1
  [tri_32] -> Relational Operator5/2
  Relational Operator5/1 -> [igbt_2], Scope4/2
  [leg_3] -> Relational Operator5/1
  [igbt_5] -> Scope2/3
  [igbt_3] -> Scope2/2
  [igbt_6] -> Scope3/1
  [igbt_1] -> Scope2/1
  Relational Operator/1 -> Scope/1, [igbt_1]
  Relational Operator1/1 -> Scope/2, [igbt_4]
  [tri_11] -> Relational Operator/2
  [leg_1] -> Relational Operator/1
  [leg_2] -> Relational Operator3/1
  [tri_22] -> Relational Operator3/2
  Relational Operator2/1 -> Scope1/1, [igbt_3]
  [leg_2] -> Relational Operator2/1
  Relational Operator3/1 -> Scope1/2, [igbt_6]
  [leg_1] -> Relational Operator1/1
  [tri_12] -> Relational Operator1/2
  [igbt_4] -> Scope3/3
  In2/1 -> [leg_2]
  In1/1 -> [leg_1]
  In3/1 -> [leg_3]
  Triangle Generator/1 -> Subsystem/1(In1)
  Subsystem/1(Out1) -> [tri_11]
  Subsystem/2(Out2) -> [tri_12]
  Triangle Generator3/1 -> Subsystem1/1(In1)
  Subsystem1/1(Out1) -> [tri_21]
  Subsystem1/2(Out2) -> [tri_22]
  Subsystem2/1(Out1) -> [tri_31]
  Subsystem2/2(Out2) -> [tri_32]
  Triangle Generator4/1 -> Subsystem2/1(In1)

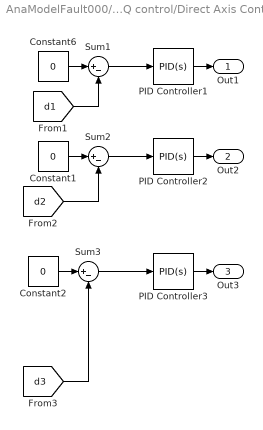
== system AnaModelFault000/Supply and control/DQ control/Direct Axis Control ==
  Constant1 : Constant  Value=0
  Constant2 : Constant  Value=0
  Constant6 : Constant  Value=0
  PID Controller1 : simulink/Continuous/PID Controller  Controller=PID  Form=Parallel  TimeDomain=Continuous-time  SampleTime=-1  IntegratorMethod=Forward Euler  FilterMethod=Forward Euler  ControllerParametersSource=internal  P=Kp  I=Ki  D=0  UseFilter=on  N=1  TunerSelectOption=Transfer Function Based (PID Tuner App)  InitialConditionSource=internal  InitialConditionForIntegrator=0  InitialConditionForFilter=0  DifferentiatorICPrevScaledInput=0  ExternalReset=none  TrackingMode=off  Kt=1  LimitOutput=off  UpperSaturationLimit=inf  LowerSaturationLimit=-inf  LinearizeAsGain=on  AntiWindupMode=none  Kb=1  POutMin=[]  POutMax=[]  IOutMin=[]  IOutMax=[]  DOutMin=[]  DOutMax=[]  NOutMin=[]  NOutMax=[]  SumOutMin=[]  SumOutMax=[]  SaturationOutMin=[]  SaturationOutMax=[]  PParamMin=[]  PParamMax=[]  IParamMin=[]  IParamMax=[]  DParamMin=[]  DParamMax=[]  NParamMin=[]  NParamMax=[]  KbParamMin=[]  KbParamMax=[]  KtParamMin=[]  KtParamMax=[]  KbOutMin=[]  KbOutMax=[]  KtOutMin=[]  KtOutMax=[]  IntegratorOutMin=[]  IntegratorOutMax=[]  FilterOutMin=[]  FilterOutMax=[]  SumI1OutMin=[]  SumI1OutMax=[]  SumI2OutMin=[]  SumI2OutMax=[]  SumI3OutMin=[]  SumI3OutMax=[]  SumI4OutMin=[]  SumI4OutMax=[]  SumDOutMin=[]  SumDOutMax=[]  DifferentiatorOutMin=[]  DifferentiatorOutMax=[]  FilterDiffOutCoefMin=[]  FilterDiffOutCoefMax=[]  ReciprocalOutMin=[]  ReciprocalOutMax=[]  SumDenOutMin=[]  SumDenOutMax=[]  SumNumOutMin=[]  SumNumOutMax=[]  DivideOutMin=[]  DivideOutMax=[]  IntegratorContinuousStateAttributes=''  IntegratorStateMustResolveToSignalObject=off  IntegratorRTWStateStorageClass=Auto  FilterContinuousStateAttributes=''  FilterStateMustResolveToSignalObject=off  FilterRTWStateStorageClass=Auto  ParallelPVariant=InternalParameters  IdealPVariant=Disabled  IVariant=InternalParameters  DVariant=InternalParameters  IntegratorVariant=Continuous  SatVariant=Disabled  AWVariant=Passthrough  PCopyVariant=Disabled  TRVariant=Disabled  FdbkBlocksVariant=Forward  IdealPFdbkVariant=Disabled  SatFdbkVariant=Disabled  DerivativeFilterVariant=ContFilter  NVariant=InternalParameters  NCopyVariant=Disabled  FilterICVariant=InternalICsFilter  IntegratorICVariant=InternalICs  ExternalResetVariant=Disabled  TRSumVariant=Passthrough  SumFdbkVariant=Disabled  SumVariant=Sum_PID
  PID Controller2 : simulink/Continuous/PID Controller  Controller=PID  Form=Parallel  TimeDomain=Continuous-time  SampleTime=-1  IntegratorMethod=Forward Euler  FilterMethod=Forward Euler  ControllerParametersSource=internal  P=Kp  I=Ki  D=0  UseFilter=on  N=1  TunerSelectOption=Transfer Function Based (PID Tuner App)  InitialConditionSource=internal  InitialConditionForIntegrator=0  InitialConditionForFilter=0  DifferentiatorICPrevScaledInput=0  ExternalReset=none  TrackingMode=off  Kt=1  LimitOutput=off  UpperSaturationLimit=inf  LowerSaturationLimit=-inf  LinearizeAsGain=on  AntiWindupMode=none  Kb=1  POutMin=[]  POutMax=[]  IOutMin=[]  IOutMax=[]  DOutMin=[]  DOutMax=[]  NOutMin=[]  NOutMax=[]  SumOutMin=[]  SumOutMax=[]  SaturationOutMin=[]  SaturationOutMax=[]  PParamMin=[]  PParamMax=[]  IParamMin=[]  IParamMax=[]  DParamMin=[]  DParamMax=[]  NParamMin=[]  NParamMax=[]  KbParamMin=[]  KbParamMax=[]  KtParamMin=[]  KtParamMax=[]  KbOutMin=[]  KbOutMax=[]  KtOutMin=[]  KtOutMax=[]  IntegratorOutMin=[]  IntegratorOutMax=[]  FilterOutMin=[]  FilterOutMax=[]  SumI1OutMin=[]  SumI1OutMax=[]  SumI2OutMin=[]  SumI2OutMax=[]  SumI3OutMin=[]  SumI3OutMax=[]  SumI4OutMin=[]  SumI4OutMax=[]  SumDOutMin=[]  SumDOutMax=[]  DifferentiatorOutMin=[]  DifferentiatorOutMax=[]  FilterDiffOutCoefMin=[]  FilterDiffOutCoefMax=[]  ReciprocalOutMin=[]  ReciprocalOutMax=[]  SumDenOutMin=[]  SumDenOutMax=[]  SumNumOutMin=[]  SumNumOutMax=[]  DivideOutMin=[]  DivideOutMax=[]  IntegratorContinuousStateAttributes=''  IntegratorStateMustResolveToSignalObject=off  IntegratorRTWStateStorageClass=Auto  FilterContinuousStateAttributes=''  FilterStateMustResolveToSignalObject=off  FilterRTWStateStorageClass=Auto  ParallelPVariant=InternalParameters  IdealPVariant=Disabled  IVariant=InternalParameters  DVariant=InternalParameters  IntegratorVariant=Continuous  SatVariant=Disabled  AWVariant=Passthrough  PCopyVariant=Disabled  TRVariant=Disabled  FdbkBlocksVariant=Forward  IdealPFdbkVariant=Disabled  SatFdbkVariant=Disabled  DerivativeFilterVariant=ContFilter  NVariant=InternalParameters  NCopyVariant=Disabled  FilterICVariant=InternalICsFilter  IntegratorICVariant=InternalICs  ExternalResetVariant=Disabled  TRSumVariant=Passthrough  SumFdbkVariant=Disabled  SumVariant=Sum_PID
  PID Controller3 : simulink/Continuous/PID Controller  Controller=PID  Form=Parallel  TimeDomain=Continuous-time  SampleTime=-1  IntegratorMethod=Forward Euler  FilterMethod=Forward Euler  ControllerParametersSource=internal  P=Kp  I=Ki  D=0  UseFilter=on  N=1  TunerSelectOption=Transfer Function Based (PID Tuner App)  InitialConditionSource=internal  InitialConditionForIntegrator=0  InitialConditionForFilter=0  DifferentiatorICPrevScaledInput=0  ExternalReset=none  TrackingMode=off  Kt=1  LimitOutput=off  UpperSaturationLimit=inf  LowerSaturationLimit=-inf  LinearizeAsGain=on  AntiWindupMode=none  Kb=1  POutMin=[]  POutMax=[]  IOutMin=[]  IOutMax=[]  DOutMin=[]  DOutMax=[]  NOutMin=[]  NOutMax=[]  SumOutMin=[]  SumOutMax=[]  SaturationOutMin=[]  SaturationOutMax=[]  PParamMin=[]  PParamMax=[]  IParamMin=[]  IParamMax=[]  DParamMin=[]  DParamMax=[]  NParamMin=[]  NParamMax=[]  KbParamMin=[]  KbParamMax=[]  KtParamMin=[]  KtParamMax=[]  KbOutMin=[]  KbOutMax=[]  KtOutMin=[]  KtOutMax=[]  IntegratorOutMin=[]  IntegratorOutMax=[]  FilterOutMin=[]  FilterOutMax=[]  SumI1OutMin=[]  SumI1OutMax=[]  SumI2OutMin=[]  SumI2OutMax=[]  SumI3OutMin=[]  SumI3OutMax=[]  SumI4OutMin=[]  SumI4OutMax=[]  SumDOutMin=[]  SumDOutMax=[]  DifferentiatorOutMin=[]  DifferentiatorOutMax=[]  FilterDiffOutCoefMin=[]  FilterDiffOutCoefMax=[]  ReciprocalOutMin=[]  ReciprocalOutMax=[]  SumDenOutMin=[]  SumDenOutMax=[]  SumNumOutMin=[]  SumNumOutMax=[]  DivideOutMin=[]  DivideOutMax=[]  IntegratorContinuousStateAttributes=''  IntegratorStateMustResolveToSignalObject=off  IntegratorRTWStateStorageClass=Auto  FilterContinuousStateAttributes=''  FilterStateMustResolveToSignalObject=off  FilterRTWStateStorageClass=Auto  ParallelPVariant=InternalParameters  IdealPVariant=Disabled  IVariant=InternalParameters  DVariant=InternalParameters  IntegratorVariant=Continuous  SatVariant=Disabled  AWVariant=Passthrough  PCopyVariant=Disabled  TRVariant=Disabled  FdbkBlocksVariant=Forward  IdealPFdbkVariant=Disabled  SatFdbkVariant=Disabled  DerivativeFilterVariant=ContFilter  NVariant=InternalParameters  NCopyVariant=Disabled  FilterICVariant=InternalICsFilter  IntegratorICVariant=InternalICs  ExternalResetVariant=Disabled  TRSumVariant=Passthrough  SumFdbkVariant=Disabled  SumVariant=Sum_PID
  Sum1 : Sum  Inputs=|+-
  Sum2 : Sum  Inputs=|+-
  Sum3 : Sum  Inputs=|+-
  Out1 : Outport
  Out2 : Outport  Port=2
  Out3 : Outport  Port=3
  wires:
  Constant1/1 -> Sum2/1
  Sum2/1 -> PID Controller2/1
  PID Controller2/1 -> Out2/1
  PID Controller1/1 -> Out1/1
  PID Controller3/1 -> Out3/1
  Sum3/1 -> PID Controller3/1
  Constant2/1 -> Sum3/1
  Constant6/1 -> Sum1/1
  Sum1/1 -> PID Controller1/1
  [d1] -> Sum1/2
  [d2] -> Sum2/2
  [d3] -> Sum3/2

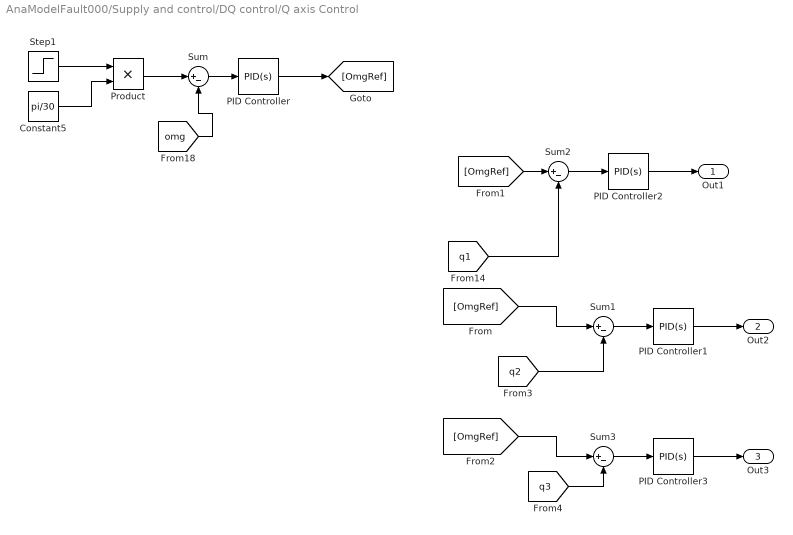
== system AnaModelFault000/Supply and control/DQ control/Q axis Control  ==
  Constant5 : Constant  Value=pi/30
  PID Controller : simulink/Continuous/PID Controller  Controller=PID  Form=Parallel  TimeDomain=Continuous-time  SampleTime=-1  IntegratorMethod=Forward Euler  FilterMethod=Forward Euler  ControllerParametersSource=internal  P=0.1  I=0.01  D=0  UseFilter=on  N=1  TunerSelectOption=Transfer Function Based (PID Tuner App)  InitialConditionSource=internal  InitialConditionForIntegrator=0  InitialConditionForFilter=0  DifferentiatorICPrevScaledInput=0  ExternalReset=none  TrackingMode=off  Kt=1  LimitOutput=off  UpperSaturationLimit=inf  LowerSaturationLimit=-inf  LinearizeAsGain=on  AntiWindupMode=none  Kb=1  POutMin=[]  POutMax=[]  IOutMin=[]  IOutMax=[]  DOutMin=[]  DOutMax=[]  NOutMin=[]  NOutMax=[]  SumOutMin=[]  SumOutMax=[]  SaturationOutMin=[]  SaturationOutMax=[]  PParamMin=[]  PParamMax=[]  IParamMin=[]  IParamMax=[]  DParamMin=[]  DParamMax=[]  NParamMin=[]  NParamMax=[]  KbParamMin=[]  KbParamMax=[]  KtParamMin=[]  KtParamMax=[]  KbOutMin=[]  KbOutMax=[]  KtOutMin=[]  KtOutMax=[]  IntegratorOutMin=[]  IntegratorOutMax=[]  FilterOutMin=[]  FilterOutMax=[]  SumI1OutMin=[]  SumI1OutMax=[]  SumI2OutMin=[]  SumI2OutMax=[]  SumI3OutMin=[]  SumI3OutMax=[]  SumI4OutMin=[]  SumI4OutMax=[]  SumDOutMin=[]  SumDOutMax=[]  DifferentiatorOutMin=[]  DifferentiatorOutMax=[]  FilterDiffOutCoefMin=[]  FilterDiffOutCoefMax=[]  ReciprocalOutMin=[]  ReciprocalOutMax=[]  SumDenOutMin=[]  SumDenOutMax=[]  SumNumOutMin=[]  SumNumOutMax=[]  DivideOutMin=[]  DivideOutMax=[]  IntegratorContinuousStateAttributes=''  IntegratorStateMustResolveToSignalObject=off  IntegratorRTWStateStorageClass=Auto  FilterContinuousStateAttributes=''  FilterStateMustResolveToSignalObject=off  FilterRTWStateStorageClass=Auto  ParallelPVariant=InternalParameters  IdealPVariant=Disabled  IVariant=InternalParameters  DVariant=InternalParameters  IntegratorVariant=Continuous  SatVariant=Disabled  AWVariant=Passthrough  PCopyVariant=Disabled  TRVariant=Disabled  FdbkBlocksVariant=Forward  IdealPFdbkVariant=Disabled  SatFdbkVariant=Disabled  DerivativeFilterVariant=ContFilter  NVariant=InternalParameters  NCopyVariant=Disabled  FilterICVariant=InternalICsFilter  IntegratorICVariant=InternalICs  ExternalResetVariant=Disabled  TRSumVariant=Passthrough  SumFdbkVariant=Disabled  SumVariant=Sum_PID
  PID Controller1 : simulink/Continuous/PID Controller  Controller=PID  Form=Parallel  TimeDomain=Continuous-time  SampleTime=-1  IntegratorMethod=Forward Euler  FilterMethod=Forward Euler  ControllerParametersSource=internal  P=Kp  I=Ki  D=0  UseFilter=on  N=1  TunerSelectOption=Transfer Function Based (PID Tuner App)  InitialConditionSource=internal  InitialConditionForIntegrator=0  InitialConditionForFilter=0  DifferentiatorICPrevScaledInput=0  ExternalReset=none  TrackingMode=off  Kt=1  LimitOutput=off  UpperSaturationLimit=inf  LowerSaturationLimit=-inf  LinearizeAsGain=on  AntiWindupMode=none  Kb=1  POutMin=[]  POutMax=[]  IOutMin=[]  IOutMax=[]  DOutMin=[]  DOutMax=[]  NOutMin=[]  NOutMax=[]  SumOutMin=[]  SumOutMax=[]  SaturationOutMin=[]  SaturationOutMax=[]  PParamMin=[]  PParamMax=[]  IParamMin=[]  IParamMax=[]  DParamMin=[]  DParamMax=[]  NParamMin=[]  NParamMax=[]  KbParamMin=[]  KbParamMax=[]  KtParamMin=[]  KtParamMax=[]  KbOutMin=[]  KbOutMax=[]  KtOutMin=[]  KtOutMax=[]  IntegratorOutMin=[]  IntegratorOutMax=[]  FilterOutMin=[]  FilterOutMax=[]  SumI1OutMin=[]  SumI1OutMax=[]  SumI2OutMin=[]  SumI2OutMax=[]  SumI3OutMin=[]  SumI3OutMax=[]  SumI4OutMin=[]  SumI4OutMax=[]  SumDOutMin=[]  SumDOutMax=[]  DifferentiatorOutMin=[]  DifferentiatorOutMax=[]  FilterDiffOutCoefMin=[]  FilterDiffOutCoefMax=[]  ReciprocalOutMin=[]  ReciprocalOutMax=[]  SumDenOutMin=[]  SumDenOutMax=[]  SumNumOutMin=[]  SumNumOutMax=[]  DivideOutMin=[]  DivideOutMax=[]  IntegratorContinuousStateAttributes=''  IntegratorStateMustResolveToSignalObject=off  IntegratorRTWStateStorageClass=Auto  FilterContinuousStateAttributes=''  FilterStateMustResolveToSignalObject=off  FilterRTWStateStorageClass=Auto  ParallelPVariant=InternalParameters  IdealPVariant=Disabled  IVariant=InternalParameters  DVariant=InternalParameters  IntegratorVariant=Continuous  SatVariant=Disabled  AWVariant=Passthrough  PCopyVariant=Disabled  TRVariant=Disabled  FdbkBlocksVariant=Forward  IdealPFdbkVariant=Disabled  SatFdbkVariant=Disabled  DerivativeFilterVariant=ContFilter  NVariant=InternalParameters  NCopyVariant=Disabled  FilterICVariant=InternalICsFilter  IntegratorICVariant=InternalICs  ExternalResetVariant=Disabled  TRSumVariant=Passthrough  SumFdbkVariant=Disabled  SumVariant=Sum_PID
  PID Controller2 : simulink/Continuous/PID Controller  Controller=PID  Form=Parallel  TimeDomain=Continuous-time  SampleTime=-1  IntegratorMethod=Forward Euler  FilterMethod=Forward Euler  ControllerParametersSource=internal  P=Kp  I=Ki  D=0  UseFilter=on  N=1  TunerSelectOption=Transfer Function Based (PID Tuner App)  InitialConditionSource=internal  InitialConditionForIntegrator=0  InitialConditionForFilter=0  DifferentiatorICPrevScaledInput=0  ExternalReset=none  TrackingMode=off  Kt=1  LimitOutput=off  UpperSaturationLimit=inf  LowerSaturationLimit=-inf  LinearizeAsGain=on  AntiWindupMode=none  Kb=1  POutMin=[]  POutMax=[]  IOutMin=[]  IOutMax=[]  DOutMin=[]  DOutMax=[]  NOutMin=[]  NOutMax=[]  SumOutMin=[]  SumOutMax=[]  SaturationOutMin=[]  SaturationOutMax=[]  PParamMin=[]  PParamMax=[]  IParamMin=[]  IParamMax=[]  DParamMin=[]  DParamMax=[]  NParamMin=[]  NParamMax=[]  KbParamMin=[]  KbParamMax=[]  KtParamMin=[]  KtParamMax=[]  KbOutMin=[]  KbOutMax=[]  KtOutMin=[]  KtOutMax=[]  IntegratorOutMin=[]  IntegratorOutMax=[]  FilterOutMin=[]  FilterOutMax=[]  SumI1OutMin=[]  SumI1OutMax=[]  SumI2OutMin=[]  SumI2OutMax=[]  SumI3OutMin=[]  SumI3OutMax=[]  SumI4OutMin=[]  SumI4OutMax=[]  SumDOutMin=[]  SumDOutMax=[]  DifferentiatorOutMin=[]  DifferentiatorOutMax=[]  FilterDiffOutCoefMin=[]  FilterDiffOutCoefMax=[]  ReciprocalOutMin=[]  ReciprocalOutMax=[]  SumDenOutMin=[]  SumDenOutMax=[]  SumNumOutMin=[]  SumNumOutMax=[]  DivideOutMin=[]  DivideOutMax=[]  IntegratorContinuousStateAttributes=''  IntegratorStateMustResolveToSignalObject=off  IntegratorRTWStateStorageClass=Auto  FilterContinuousStateAttributes=''  FilterStateMustResolveToSignalObject=off  FilterRTWStateStorageClass=Auto  ParallelPVariant=InternalParameters  IdealPVariant=Disabled  IVariant=InternalParameters  DVariant=InternalParameters  IntegratorVariant=Continuous  SatVariant=Disabled  AWVariant=Passthrough  PCopyVariant=Disabled  TRVariant=Disabled  FdbkBlocksVariant=Forward  IdealPFdbkVariant=Disabled  SatFdbkVariant=Disabled  DerivativeFilterVariant=ContFilter  NVariant=InternalParameters  NCopyVariant=Disabled  FilterICVariant=InternalICsFilter  IntegratorICVariant=InternalICs  ExternalResetVariant=Disabled  TRSumVariant=Passthrough  SumFdbkVariant=Disabled  SumVariant=Sum_PID
  PID Controller3 : simulink/Continuous/PID Controller  Controller=PID  Form=Parallel  TimeDomain=Continuous-time  SampleTime=-1  IntegratorMethod=Forward Euler  FilterMethod=Forward Euler  ControllerParametersSource=internal  P=Kp  I=Ki  D=0  UseFilter=on  N=1  TunerSelectOption=Transfer Function Based (PID Tuner App)  InitialConditionSource=internal  InitialConditionForIntegrator=0  InitialConditionForFilter=0  DifferentiatorICPrevScaledInput=0  ExternalReset=none  TrackingMode=off  Kt=1  LimitOutput=off  UpperSaturationLimit=inf  LowerSaturationLimit=-inf  LinearizeAsGain=on  AntiWindupMode=none  Kb=1  POutMin=[]  POutMax=[]  IOutMin=[]  IOutMax=[]  DOutMin=[]  DOutMax=[]  NOutMin=[]  NOutMax=[]  SumOutMin=[]  SumOutMax=[]  SaturationOutMin=[]  SaturationOutMax=[]  PParamMin=[]  PParamMax=[]  IParamMin=[]  IParamMax=[]  DParamMin=[]  DParamMax=[]  NParamMin=[]  NParamMax=[]  KbParamMin=[]  KbParamMax=[]  KtParamMin=[]  KtParamMax=[]  KbOutMin=[]  KbOutMax=[]  KtOutMin=[]  KtOutMax=[]  IntegratorOutMin=[]  IntegratorOutMax=[]  FilterOutMin=[]  FilterOutMax=[]  SumI1OutMin=[]  SumI1OutMax=[]  SumI2OutMin=[]  SumI2OutMax=[]  SumI3OutMin=[]  SumI3OutMax=[]  SumI4OutMin=[]  SumI4OutMax=[]  SumDOutMin=[]  SumDOutMax=[]  DifferentiatorOutMin=[]  DifferentiatorOutMax=[]  FilterDiffOutCoefMin=[]  FilterDiffOutCoefMax=[]  ReciprocalOutMin=[]  ReciprocalOutMax=[]  SumDenOutMin=[]  SumDenOutMax=[]  SumNumOutMin=[]  SumNumOutMax=[]  DivideOutMin=[]  DivideOutMax=[]  IntegratorContinuousStateAttributes=''  IntegratorStateMustResolveToSignalObject=off  IntegratorRTWStateStorageClass=Auto  FilterContinuousStateAttributes=''  FilterStateMustResolveToSignalObject=off  FilterRTWStateStorageClass=Auto  ParallelPVariant=InternalParameters  IdealPVariant=Disabled  IVariant=InternalParameters  DVariant=InternalParameters  IntegratorVariant=Continuous  SatVariant=Disabled  AWVariant=Passthrough  PCopyVariant=Disabled  TRVariant=Disabled  FdbkBlocksVariant=Forward  IdealPFdbkVariant=Disabled  SatFdbkVariant=Disabled  DerivativeFilterVariant=ContFilter  NVariant=InternalParameters  NCopyVariant=Disabled  FilterICVariant=InternalICsFilter  IntegratorICVariant=InternalICs  ExternalResetVariant=Disabled  TRSumVariant=Passthrough  SumFdbkVariant=Disabled  SumVariant=Sum_PID
  Product : Product
  Step1 : Step  Time=0.02  After=3500  SampleTime=0
  Sum{,1..3} (4 alike) : Sum  Inputs=|+-
  Out1 : Outport
  Out2 : Outport  Port=2
  Out3 : Outport  Port=3
  wires:
  Step1/1 -> Product/1
  Sum/1 -> PID Controller/1
  Sum2/1 -> PID Controller2/1
  PID Controller/1 -> [OmgRef]
  [omg] -> Sum/2
  Constant5/1 -> Product/2
  Product/1 -> Sum/1
  PID Controller2/1 -> Out1/1
  PID Controller1/1 -> Out2/1
  [OmgRef] -> Sum1/1
  Sum1/1 -> PID Controller1/1
  Sum3/1 -> PID Controller3/1
  [OmgRef] -> Sum3/1
  PID Controller3/1 -> Out3/1
  [q1] -> Sum2/2
  [q2] -> Sum1/2
  [q3] -> Sum3/2
  [OmgRef] -> Sum2/1

== system AnaModelFault000/Supply and control/Inverter Phase 2/Low-Pass Filter2 ==
  Ground4 : powerlib/Elements/Ground  LConnTagsString=a
      settings: SourceProductName=Simscape Electrical
  Series RLC Branch4 : powerlib/Elements/Series RLC Branch  LConnTagsString=__new0  RConnTagsString=__new0  BranchType=C  Resistance=1000  Inductance=3e-3  SetiL0=off  InitialCurrent=0  Capacitance=150e-6  Setx0=off  InitialVoltage=0  Measurements=None
      settings: SourceProductName=Simscape Electrical
  Series RLC Branch5 : powerlib/Elements/Series RLC Branch  LConnTagsString=__new0  RConnTagsString=__new0  BranchType=RL  Resistance=18  Inductance=25e-3  SetiL0=off  InitialCurrent=0  Capacitance=1e-6  Setx0=off  InitialVoltage=0  Measurements=None
      settings: SourceProductName=Simscape Electrical
  + : PMIOPort  Side=Right
  - : PMIOPort  Port=2  Side=Right
  In : PMIOPort  Port=3  Side=Left
  connections:
  Series RLC Branch5/LConn1 -- In/RConn1
  -/RConn1 -- Ground4/LConn1 -- Series RLC Branch4/RConn1
  +/RConn1 -- Series RLC Branch4/LConn1 -- Series RLC Branch5/RConn1

== system AnaModelFault000/Supply and control/Inverter Phase 3/Low-Pass Filter2 ==
  Ground4 : powerlib/Elements/Ground  LConnTagsString=a
      settings: SourceProductName=Simscape Electrical
  Series RLC Branch4 : powerlib/Elements/Series RLC Branch  LConnTagsString=__new0  RConnTagsString=__new0  BranchType=C  Resistance=1000  Inductance=3e-3  SetiL0=off  InitialCurrent=0  Capacitance=150e-6  Setx0=off  InitialVoltage=0  Measurements=None
      settings: SourceProductName=Simscape Electrical
  Series RLC Branch5 : powerlib/Elements/Series RLC Branch  LConnTagsString=__new0  RConnTagsString=__new0  BranchType=RL  Resistance=18  Inductance=25e-3  SetiL0=off  InitialCurrent=0  Capacitance=1e-6  Setx0=off  InitialVoltage=0  Measurements=None
      settings: SourceProductName=Simscape Electrical
  + : PMIOPort  Side=Right
  - : PMIOPort  Port=2  Side=Right
  In : PMIOPort  Port=3  Side=Left
  connections:
  Series RLC Branch5/RConn1 -- Series RLC Branch4/LConn1 -- +/RConn1
  Series RLC Branch4/RConn1 -- Ground4/LConn1 -- -/RConn1
  Series RLC Branch5/LConn1 -- In/RConn1

== system AnaModelFault000/Supply and control/PWM Switching Signals for Phase 2/Subsystem ==
  In1 : Inport
  Constant : Constant  Value=0.5
  Product : Product
  Sum : Sum  Inputs=|++
  Sum1 : Sum  Inputs=|+-
  Out1 : Outport
  Out2 : Outport  Port=2
  wires:
  Sum1/1 -> Out2/1
  Sum/1 -> Out1/1
  Constant/1 -> Sum1/2, Sum/2, Product/2
  In1/1 -> Product/1
  Product/1 -> Sum1/1, Sum/1

== system AnaModelFault000/Supply and control/PWM Switching Signals for Phase 2/Subsystem1 ==
  In1 : Inport
  Constant : Constant  Value=0.5
  Product : Product
  Sum : Sum  Inputs=|++
  Sum1 : Sum  Inputs=|+-
  Out1 : Outport
  Out2 : Outport  Port=2
  wires:
  Product/1 -> Sum/1, Sum1/1
  In1/1 -> Product/1
  Constant/1 -> Product/2, Sum/2, Sum1/2
  Sum/1 -> Out1/1
  Sum1/1 -> Out2/1

== system AnaModelFault000/Supply and control/PWM Switching Signals for Phase 2/Subsystem2 ==
  In1 : Inport
  Constant : Constant  Value=0.5
  Product : Product
  Sum : Sum  Inputs=|++
  Sum1 : Sum  Inputs=|+-
  Out1 : Outport
  Out2 : Outport  Port=2
  wires:
  Sum1/1 -> Out2/1
  Sum/1 -> Out1/1
  Constant/1 -> Sum1/2, Sum/2, Product/2
  In1/1 -> Product/1
  Product/1 -> Sum1/1, Sum/1
